simulink model "Motor_CD"  (R2020a)
settings: Solver=VariableStepAuto  StartTime=0.0  StopTime=5  RelTol=1e-3
values from neighbouring files (symbols this model uses):
  A = [-3, 2, 0 ... (first row only)    [AsesoriaP3.m]    (also in Circ_Doble_Malla_ODE_plot.m = [0, 1/C2; -1/(R1*C1*R2), -(C2*R1+C2*R2+R1*C1)/(C1*C2*R1*R2)]; ControlThis_P1.m = [-1,-3,0; Controlador_Retro_plot.m = [0, 0, 1, 0; Engranes_ODE_plot.m = [0, 1; -K./(Jm2 + Jm1.*(n2./n1)^2), -B/(Jm2 + Jm1.*(n2./n1)^)
  B = [2, 0 ... (first row only)    [AsesoriaP3.m]    (also in Circ_Doble_Malla_ODE_plot.m = [0; 1/(C1*R1*R2)]; ControlThis_P1.m = [2,4,2; Controlador_Retro_plot.m = [0; Engranes_ODE_plot.m = [0; -1/(n1.*Jm2/2 + n2.*Jm1./n1)])
  F = 1 / (C*(-A-B*K)^-1*B)    [Controlador_Retro_plot.m]    (also in Ex3_ej1.m = 1 / ( C*inv( -A-B*K ) * B ); LQR_motor_cd_plot.m = 1 / ( C*inv( -A-B*K ) * B ); PendInv_LQR_plot.m = 1/(C*(-A-B*K)^-1*B); Tarea_21.m = 1/(C*inv(-A-B*K)*B))
  K = -[0, 0, 0, 1]*Mc^-1*H    [Controlador_Retro_plot.m]    (also in Engranes_ODE_plot.m = 0.8; Ex3_ej1.m = -[0 0 0 1]*inv(Mc)*H; LQR_motor_cd_plot.m = lqr(A,B,Q,R); PendInv_LQR_plot.m = lqr(A,B,Q,R))
undefined symbols (not defined in the file or in its folder): p
libraries: simulink x1
settings Model: Creator=luis  LastModifiedBy=micro microndas

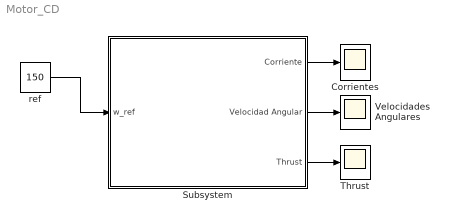
== system Motor_CD ==
  "Corrientes " : Scope
  Subsystem : Subsystem
  Thrust : Scope
  "Velocidades Angulares " : Scope
  ref : Constant  Value=150
  wires:
  ref/1 -> Subsystem/1(w_ref)
  Subsystem/3(Thrust) -> Thrust/1
  Subsystem/2(Velocidad Angular) -> "Velocidades Angulares "/1
  Subsystem/1(Corriente) -> "Corrientes "/1

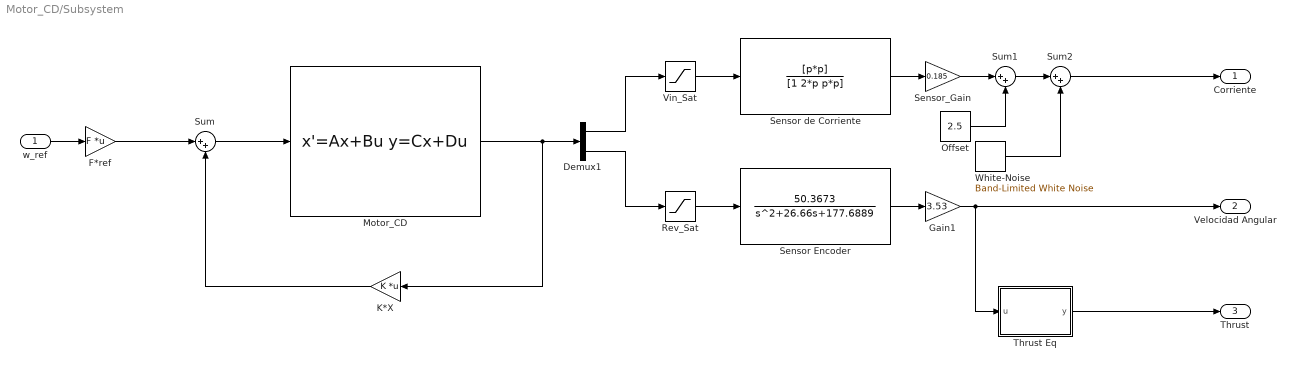
== system Motor_CD/Subsystem ==
  w_ref : Inport
  Demux1 : Demux  Outputs=2
  F*ref : Gain  Gain=F  Multiplication=Matrix(K*u)
  Gain1 : Gain  Gain=3.53
  K*X : Gain  Gain=K  Multiplication=Matrix(K*u)
  Motor_CD : StateSpace  A=A  B=B  C=eye(2)  D=[0;0]  InitialCondition=0  ContinuousStateAttributes={'i_t', 'w_t'}
  Offset : Constant  Value=2.5
  Rev_Sat : Saturate  UpperLimit=7500  LowerLimit=0
  Sensor Encoder : TransferFcn  Numerator=[50.3673]  Denominator=[1 26.66 177.6889]  ContinuousStateAttributes='Position'
  "Sensor de Corriente " : TransferFcn  Numerator=[p*p]  Denominator=[1 2*p p*p]  ContinuousStateAttributes='Corriente'
  Sensor_Gain : Gain  Gain=0.185
  Sum : Sum  Inputs=|++
  Sum1 : Sum  Inputs=|++
  Sum2 : Sum  Inputs=|++
  Thrust Eq : MATLAB Function  TreatAsAtomicUnit=on
  Vin_Sat : Saturate  UpperLimit=5  LowerLimit=-5
  White-Noise : simulink/Sources/Band-Limited White Noise  Cov=[1e-8]  Ts=0.001  seed=[23341]
  Corriente : Outport
  Velocidad Angular : Outport  Port=2
  Thrust : Outport  Port=3
  wires:
  Rev_Sat/1 -> Sensor Encoder/1
  "Sensor de Corriente "/1 -> Sensor_Gain/1
  Demux1/2 -> Rev_Sat/1
  Gain1/1 -> Velocidad Angular/1, Thrust Eq/1(u)
  Sum1/1 -> Sum2/1
  K*X/1 -> Sum/2
  Demux1/1 -> Vin_Sat/1
  Motor_CD/1 -> K*X/1, Demux1/1
  White-Noise/1 -> Sum2/2
  Thrust Eq/1(y) -> Thrust/1
  Sum/1 -> Motor_CD/1
  Offset/1 -> Sum1/2
  F*ref/1 -> Sum/1
  Sum2/1 -> Corriente/1
  Sensor_Gain/1 -> Sum1/1
  Sensor Encoder/1 -> Gain1/1
  Vin_Sat/1 -> "Sensor de Corriente "/1
  w_ref/1 -> F*ref/1

== matlab function Motor_CD/Subsystem/Thrust Eq ==
  data: u input; y output
function y = Thrust_Eq(u)

% Valores para propela
    % Thrust = Thrust_Coef*( density*Rev*Rev*Diam*Diam*Diam*Diam )

    Thrust_Coef = 0.014;
    density = 1e3; %kg/mts*mts*mts
    Diam = 1.0; %mts
    
y = ( Thrust_Coef )*( density )*( u^2 )*( Diam^4 ) ;
